simulink model "PV_ESS_MPC_Switching_Template"  (R2025a)
settings: Solver=ode3  StartTime=0.0  StopTime=0.01  FixedStep=Ts_power  RelTol=1e-3
PreLoadFcn:
  | addpath('D:/PV_MPPT/PV_ESS_MPC_Paper_Reproduction/scripts');
model workspace (MAT data in the model file):
  Battery_blocking = 1
  Battery_connect = 0
  Cdc = 0.006
  Cf = 0.001338
  Cpv = 0.005
  Db0 = 0.75
  Db_max = 0.95
  Db_min = 0.05
  Dpv0 = 0.544166666667
  Dpv_max = 0.75
  Dpv_min = 0.35
  Dpv_off_mppt = 0.46
  Dpv_step = 0.0002
  Fsw_bat = 5000
  Fsw_pv = 5000
  G_profile = timeseries
  G_profile.Name = 'unnamed'
  G_profile.DataInfo = tsdata.datametadata
  G_profile.DataInfo.Interpolation = tsdata.interpolation
  G_profile.DataInfo.Interpolation.Fhandle : function handle (value not decoded)
  G_profile.DataInfo.Interpolation.Name = 'linear'
  G_profile.TimeInfo = tsdata.timemetadata
  G_profile.TimeInfo.Length = 5
  G_profile.TimeInfo.DuplicateTimes = 0
  G_profile.TimeInfo.Time_ = [0; 1; 2; 3; 4]
  G_profile.TimeInfo.Initialized = 1
  G_profile.QualityInfo = tsdata.qualmetadata
  G_profile.Data_ = [400; 400; 800; 800; 400]
  GridVpu_profile = timeseries
  GridVpu_profile.Name = 'unnamed'
  GridVpu_profile.DataInfo = tsdata.datametadata
  GridVpu_profile.DataInfo.Interpolation = tsdata.interpolation
  GridVpu_profile.DataInfo.Interpolation.Fhandle : function handle (value not decoded)
  GridVpu_profile.DataInfo.Interpolation.Name = 'linear'
  GridVpu_profile.TimeInfo = tsdata.timemetadata
  GridVpu_profile.TimeInfo.Length = 3
  GridVpu_profile.TimeInfo.DuplicateTimes = 0
  GridVpu_profile.TimeInfo.Time_ = [0; 3.5; 3.500002]
  GridVpu_profile.TimeInfo.Initialized = 1
  GridVpu_profile.QualityInfo = tsdata.qualmetadata
  GridVpu_profile.Data_ = [1; 1; 0.9]
  ILpv0 = 0
  Ibat0 = 0
  Ibat_max = 1666.66666667
  Inverter_connect = 0
  Inverter_enable = 0
  Ki_dc = 200000
  Kii_bat = 0.02
  Kiv_bat = 100
  Kp_dc = 2500
  Kpi_bat = 0.0002
  Kpv_bat = 2
  L_grid_lv = 0.0001
  Lbat = 0.0005
  Lf = 0.0006
  Lpv = 0.0002
  Np_pv = 656
  Ns_pv = 10
  PV_blocking = 1
  PV_connect = 0
  PV_module = 'SunPower SPR-305E-WHT-D'
  P_ac_base = 500000
  P_ac_step = 500000
  P_base_mpc = 2000000
  P_bat_rated = 500000
  P_dc_1 = 600000
  P_dc_2 = 1000000
  P_pv_stc = 2000000
  Pref_max = 2200000
  Pref_min = -2200000
  Q_base_mpc = 1000000
  Q_bat_Ah = 1300
  RLbat = 0.002
  RLpv = 0.002
  R_bat_internal = 0.02
  R_grid_lv = 0.01
  Rdc1_profile = timeseries
  Rdc1_profile.Name = 'unnamed'
  Rdc1_profile.DataInfo = tsdata.datametadata
  Rdc1_profile.DataInfo.Interpolation = tsdata.interpolation
  Rdc1_profile.DataInfo.Interpolation.Fhandle : function handle (value not decoded)
  Rdc1_profile.DataInfo.Interpolation.Name = 'linear'
  Rdc1_profile.TimeInfo = tsdata.timemetadata
  Rdc1_profile.TimeInfo.Length = 3
  Rdc1_profile.TimeInfo.DuplicateTimes = 0
  Rdc1_profile.TimeInfo.Time_ = [0; 1; 1.000002]
  Rdc1_profile.TimeInfo.Initialized = 1
  Rdc1_profile.QualityInfo = tsdata.qualmetadata
  Rdc1_profile.Data_ = [1000000; 1000000; 2.4]
  Rdc2_profile = timeseries
  Rdc2_profile.Name = 'unnamed'
  Rdc2_profile.DataInfo = tsdata.datametadata
  Rdc2_profile.DataInfo.Interpolation = tsdata.interpolation
  Rdc2_profile.DataInfo.Interpolation.Fhandle : function handle (value not decoded)
  Rdc2_profile.DataInfo.Interpolation.Name = 'linear'
  Rdc2_profile.TimeInfo = tsdata.timemetadata
  Rdc2_profile.TimeInfo.Length = 5
  Rdc2_profile.TimeInfo.DuplicateTimes = 0
  Rdc2_profile.TimeInfo.Time_ = [0; 2.5; 2.500002; 3; 3.000002]
  Rdc2_profile.TimeInfo.Initialized = 1
  Rdc2_profile.QualityInfo = tsdata.qualmetadata
  Rdc2_profile.Data_ = [1000000; 1000000; 1.44; 1.44; 1000000]
  Rf = 0.019
  Ron_switch = 0.001
  SOC0 = 50
  SOC_max = 90
  SOC_min = 10
  S_sc_grid = 47000000
  S_tr = 2500000
  T_ac_step = 0.5
  T_dc_1 = 1
  T_dc_2_off = 3
  T_dc_2_on = 2.5
  T_grid_connect = 1.6
  T_grid_dip = 3.5
  T_pv_ramp_down = 3
  T_pv_ramp_up = 1
  T_sync = 1.4
  Ts_bat_ctrl = 0.0001
  Ts_mpc = 5e-05
  Ts_mppt = 0.001
  Ts_power = 2e-06
  V_bat_nom = 300
  V_tr_hv = 25000
  V_tr_lv = 690
  Vac_ll = 690
  Vdc0 = 1200
  Vdc_ref = 1200
  Vf_diode = 1
  Vpv0 = 547
  XR_grid = 10
  f_grid = 50
  lambda_sw = 0.002
  m_var = 4000000
undefined symbols (not defined in the file): DiscIntNeverNeededParam, Ion, Lithium
libraries: spsBreakerLib x5, spsCurrentMeasurementLib x4, spsThreePhaseParallelRLCLoadLib x3, spsThreePhaseVIMeasurementLib x3, spsThreePhaseBreakerLib x2, spsPWMGeneratorDCDCLib x2, spsParallelRLCBranchLib x2, spsVariableResistorLib x2, spsSeriesRLCBranchLib x2, spsVoltageMeasurementLib x2, spsBatteryLib x1, spsTwoQuadrantDCDCConverterLib x1
settings Model: Creator=Limingyu  LastModifiedBy=Limingyu
settings DataIOCC: SignalLogging=off

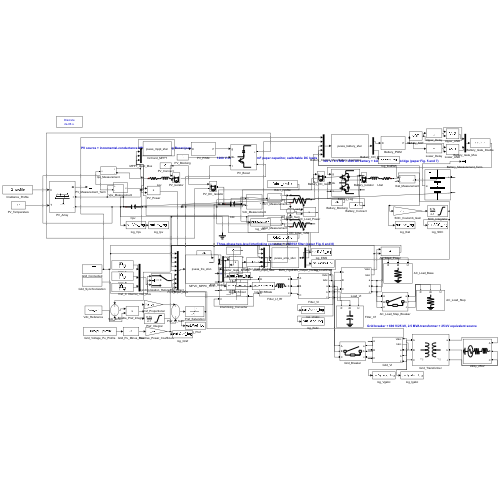
[thumbnail: Simulink's stored preview of the top-level diagram]
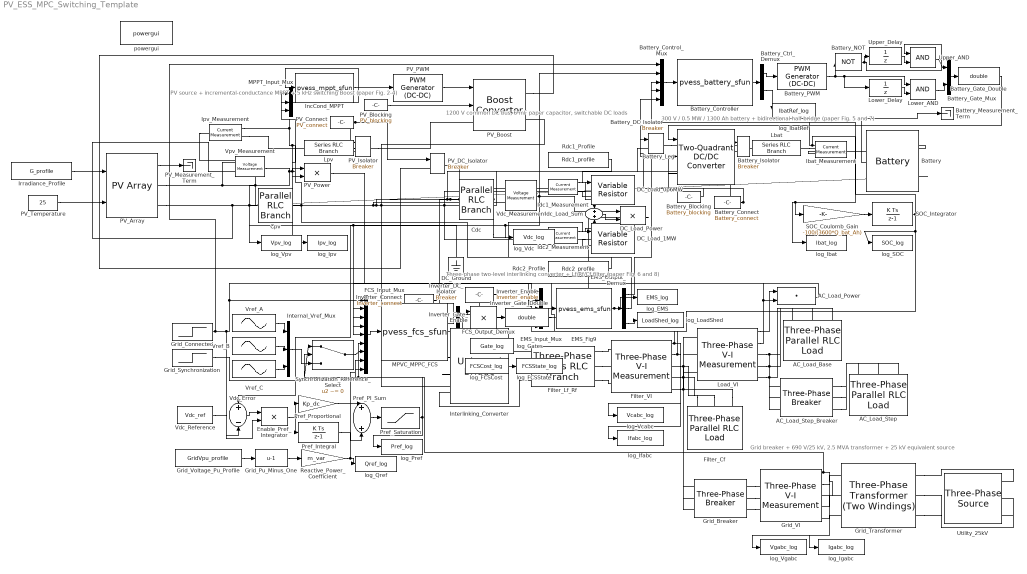
== system PV_ESS_MPC_Switching_Template ==
  note: PV source + incremental-conductance MPPT + 5 kHz switching Boost (paper Fig. 2-4)
  note: 1200 V common DC bus, 6 mF paper capacitor, switchable DC loads
  note: 300 V / 0.5 MW / 1300 Ah battery + bidirectional half bridge (paper Fig. 5 and 7)
  note: Three-phase two-level interlinking converter + Lf/Rf/Cf filter (paper Fig. 6 and 8)
  note: Grid breaker + 690 V/25 kV, 2.5 MVA transformer + 25 kV equivalent source
  AC_Load_Base : spsThreePhaseParallelRLCLoadLib/Three-Phase Parallel RLC Load  LConnTagsString=A|B|C  Configuration=Y (grounded)  NominalVoltage=Vac_ll  Vabc=[1e3 1e3 1e3]  Vabcp=[1e3 1e3 1e3]  NominalFrequency=f_grid  UnbalancedPower=off  ActivePower=P_ac_base  InductivePower=0  CapacitivePower=0  Pabc=[10e3 9e3 11e3]  QLabc=[100 90 110]  QCabc=[100 90 110]  Pabcp=[10e3 9e3 11e3]  QLabcp=[100 90 110]  QCabcp=[100 90 110]  Measurements=None  LoadType=constant Z
  AC_Load_Power : DotProduct  OutDataTypeStr=Inherit: Inherit via internal rule
  AC_Load_Step : spsThreePhaseParallelRLCLoadLib/Three-Phase Parallel RLC Load  LConnTagsString=A|B|C  Configuration=Y (grounded)  NominalVoltage=Vac_ll  Vabc=[1e3 1e3 1e3]  Vabcp=[1e3 1e3 1e3]  NominalFrequency=f_grid  UnbalancedPower=off  ActivePower=P_ac_step  InductivePower=0  CapacitivePower=0  Pabc=[10e3 9e3 11e3]  QLabc=[100 90 110]  QCabc=[100 90 110]  Pabcp=[10e3 9e3 11e3]  QLabcp=[100 90 110]  QCabcp=[100 90 110]  Measurements=None  LoadType=constant Z
  AC_Load_Step_Breaker : spsThreePhaseBreakerLib/Three-Phase Breaker  InitialState=open  SwitchA=on  SwitchB=on  SwitchC=on  SwitchTimes=T_ac_step  External=off  BreakerResistance=1e-3  SnubberResistance=1e6  SnubberCapacitance=inf  Measurements=None
  Battery : spsBatteryLib/Battery  BatType=Lithium-Ion  NomV=V_bat_nom  NomQ=Q_bat_Ah  SOC=SOC0  Batt_Tr=1  PresetModel=off  MaxQ=Q_bat_Ah  MinV=270  FullV=330  Dis_rate=650  R=R_bat_internal  Normal_OP=1170  expZone=[315,65]
  Battery_Blocking : Constant  Value=Battery_blocking
  Battery_Connect : Constant  Value=Battery_connect
  Battery_Control_Mux : Mux  Inputs=5
  Battery_Controller : M-S-Function  FunctionName=pvess_battery_sfun  Parameters=Ts_bat_ctrl,Vdc_ref,SOC_min,SOC_max,Ibat_max,Kpv_bat,Kiv_bat,Kpi_bat,Kii_bat,V_bat_nom,Db_min,Db_max
  Battery_Ctrl_Demux : Demux  Outputs=[1 1]
  Battery_DC_Isolator : spsBreakerLib/Breaker  InitialState=1  SwitchingTimes="[1/60  5/60]"  External=on  BreakerResistance=1e-3  SnubberResistance=1e6  SnubberCapacitance=inf  Measurements=None  MoreParameters=on  NoBreakLoop=off
  Battery_Gate_Double : DataTypeConversion  OutDataTypeStr=double  SaturateOnIntegerOverflow=off  RndMeth=Floor
  Battery_Gate_Mux : Mux  Inputs=2
  Battery_Isolator : spsBreakerLib/Breaker  InitialState=1  SwitchingTimes="[1/60  5/60]"  External=on  BreakerResistance=1e-3  SnubberResistance=1e6  SnubberCapacitance=inf  Measurements=None  MoreParameters=on  NoBreakLoop=off
  Battery_Leg : spsTwoQuadrantDCDCConverterLib/Two-Quadrant DC//DC Converter  ModelType=Switching devices  Ron=Ron_switch  Rs=1e6  Cs=inf  Vforward=[0,0]  Ron_Diode=Ron_switch  Rs_Diode=1e6  Cs_Diode=inf  Vf_Diode=0  Rs_CurrentSource=inf  Ron_ACsource=1e-3
  Battery_Measurement_Term : Terminator
  Battery_NOT : Logic  Operator=NOT  AllPortsSameDT=off  OutDataTypeStr=boolean
  Battery_PWM : spsPWMGeneratorDCDCLib/PWM Generator (DC-DC)  Fsw=Fsw_bat  Ts=Ts_power
  Cdc : spsParallelRLCBranchLib/Parallel RLC Branch  LConnTagsString=a  RConnTagsString=__new0  BranchType=C  Resistance=1  Inductance=1e-3  SetiL0=off  InitialCurrent=0  Capacitance=Cdc  Setx0=on  InitialVoltage=Vdc0  Measurements=None
  Cpv : spsParallelRLCBranchLib/Parallel RLC Branch  LConnTagsString=a  RConnTagsString=__new0  BranchType=C  Resistance=1  Inductance=1e-3  SetiL0=off  InitialCurrent=0  Capacitance=Cpv  Setx0=on  InitialVoltage=Vpv0  Measurements=None
  DC_Ground : spsGroundLib/Ground  LConnTagsString=a
  DC_Load_0p6MW : spsVariableResistorLib/Variable Resistor  Rabsmin=0.2
  DC_Load_1MW : spsVariableResistorLib/Variable Resistor  Rabsmin=0.2
  DC_Load_Power : Product
  EMS_Fig9 : M-S-Function  FunctionName=pvess_ems_sfun  Parameters=SOC_min,SOC_max
  EMS_Input_Mux : Mux  Inputs=5
  EMS_Output_Demux : Demux  Outputs=3
  Enable_Pref_Integrator : Product
  FCS_Input_Mux : Mux  Inputs=9
  FCS_Output_Demux : Demux  Outputs=[6 1 1]
  Filter_Cf : spsThreePhaseParallelRLCLoadLib/Three-Phase Parallel RLC Load  LConnTagsString=A|B|C  Configuration=Y (grounded)  NominalVoltage=Vac_ll  Vabc=[1e3 1e3 1e3]  Vabcp=[1e3 1e3 1e3]  NominalFrequency=f_grid  UnbalancedPower=off  ActivePower=0  InductivePower=0  CapacitivePower=2*pi*f_grid*Cf*Vac_ll^2  Pabc=[10e3 9e3 11e3]  QLabc=[100 90 110]  QCabc=[100 90 110]  Pabcp=[10e3 9e3 11e3]  QLabcp=[100 90 110]  QCabcp=[100 90 110]  Measurements=None  LoadType=constant Z
  Filter_Lf_Rf : spsThreePhaseSeriesRLCBranchLib/Three-Phase Series RLC Branch  LConnTagsString=A|B|C  RConnTagsString=A|B|C  BranchType=RL  Resistance=Rf  Inductance=Lf  Capacitance=1e-6  Measurements=None
  Filter_VI : spsThreePhaseVIMeasurementLib/Three-Phase V-I Measurement  VoltageMeasurement=phase-to-ground  SetLabelV=off  LabelV=Vabc  Vpu=off  VpuLL=off  CurrentMeasurement=yes  SetLabelI=off  LabelI=Iabc  Ipu=off  Pbase=100e6  Vbase=500e3  OutputType=Complex  PhasorSimulation=off  PSBequivalent=0
  Grid_Breaker : spsThreePhaseBreakerLib/Three-Phase Breaker  InitialState=open  SwitchA=on  SwitchB=on  SwitchC=on  SwitchTimes=T_grid_connect  External=off  BreakerResistance=1e-3  SnubberResistance=1e6  SnubberCapacitance=inf  Measurements=None
  Grid_Connected : Step  Time=T_grid_connect  SampleTime=Ts_mpc
  Grid_Pu_Minus_One : Bias  Bias=-1  SaturateOnIntegerOverflow=off
  Grid_Synchronization : Step  Time=T_sync  SampleTime=Ts_mpc
  Grid_Transformer : spsThreePhaseTransformerTwoWindingsLib/Three-Phase Transformer (Two Windings)  Winding1Connection=Yg  Winding2Connection=Yg  CoreType=Three single-phase transformers  SetSaturation=off  Hysteresis=off  DataFile='hysteresis'  SetInitialFlux=off  Measurements=None  UNITS=pu  NominalPower=[S_tr,f_grid]  Winding1=[V_tr_lv,0.002,0.06]  Winding2=[V_tr_hv,0.002,0.06]  Rm=500  Lm=500  L0=0.5  Saturation=[ 0,0 ; 0.0024,1.2 ; 1.0,1.52 ]  InitialFluxes=[ 0.8 , -0.8 , 0.7 ]  BreakLoop=off  DiscreteSolver=Trapezoidal iterative  DataType=off  TransfoNumber=1
  Grid_VI : spsThreePhaseVIMeasurementLib/Three-Phase V-I Measurement  VoltageMeasurement=phase-to-ground  SetLabelV=off  LabelV=Vabc  Vpu=off  VpuLL=off  CurrentMeasurement=yes  SetLabelI=off  LabelI=Iabc  Ipu=off  Pbase=100e6  Vbase=500e3  OutputType=Complex  PhasorSimulation=off  PSBequivalent=0
  Grid_Voltage_Pu_Profile : FromWorkspace  VariableName=GridVpu_profile
  Ibat_Measurement : spsCurrentMeasurementLib/Current Measurement  PhasorSimulation=off  OutputType=Complex  PSBequivalent=0
  Idc1_Measurement : spsCurrentMeasurementLib/Current Measurement  PhasorSimulation=off  OutputType=Complex  PSBequivalent=0
  Idc2_Measurement : spsCurrentMeasurementLib/Current Measurement  PhasorSimulation=off  OutputType=Complex  PSBequivalent=0
  Idc_Load_Sum : Sum
  IncCond_MPPT : M-S-Function  FunctionName=pvess_mppt_sfun  Parameters=Ts_mppt,Dpv0,Dpv_min,Dpv_max,Dpv_step,Dpv_off_mppt
  Interlinking_Converter : spsUniversalBridgeLib/Universal Bridge  Arms=3  SnubberResistance=1e5  SnubberCapacitance=inf  Device=IGBT / Diodes  Ron=Ron_switch  Lon=0  ForwardVoltages=[Vf_diode,Vf_diode]  ForwardVoltage=0  GTOparameters=[ 10e-6 , 20e-6 ]  IGBTparameters=[ 1e-6 , 2e-6 ]  Measurements=None  Measurements_2=None  converterType=Rectifier
  Internal_Vref_Mux : Mux  Inputs=3
  Inverter_Connect : Constant  Value=Inverter_connect
  Inverter_DC_Isolator : spsBreakerLib/Breaker  InitialState=1  SwitchingTimes="[1/60  5/60]"  External=on  BreakerResistance=1e-3  SnubberResistance=1e6  SnubberCapacitance=inf  Measurements=None  MoreParameters=on  NoBreakLoop=off
  Inverter_Enable : Constant  Value=Inverter_enable
  Inverter_Gate_Double : DataTypeConversion  OutDataTypeStr=double  SaturateOnIntegerOverflow=off  RndMeth=Floor
  Inverter_Gate_Enable : Product
  Ipv_Measurement : spsCurrentMeasurementLib/Current Measurement  PhasorSimulation=off  OutputType=Complex  PSBequivalent=0
  Irradiance_Profile : FromWorkspace  VariableName=G_profile
  Lbat : spsSeriesRLCBranchLib/Series RLC Branch  LConnTagsString=__new0  RConnTagsString=__new0  BranchType=RL  Resistance=RLbat  Inductance=Lbat  SetiL0=on  InitialCurrent=Ibat0  Capacitance=1e-6  Setx0=off  InitialVoltage=0  Measurements=None
  Load_VI : spsThreePhaseVIMeasurementLib/Three-Phase V-I Measurement  VoltageMeasurement=phase-to-ground  SetLabelV=off  LabelV=Vabc  Vpu=off  VpuLL=off  CurrentMeasurement=yes  SetLabelI=off  LabelI=Iabc  Ipu=off  Pbase=100e6  Vbase=500e3  OutputType=Complex  PhasorSimulation=off  PSBequivalent=0
  Lower_AND : Logic  AllPortsSameDT=off  OutDataTypeStr=boolean
  Lower_Delay : UnitDelay  SampleTime=Ts_power  HasFrameUpgradeWarning=on
  Lpv : spsSeriesRLCBranchLib/Series RLC Branch  LConnTagsString=__new0  RConnTagsString=__new0  BranchType=RL  Resistance=RLpv  Inductance=Lpv  SetiL0=on  InitialCurrent=ILpv0  Capacitance=1e-6  Setx0=off  InitialVoltage=0  Measurements=None
  MPPT_Input_Mux : Mux  Inputs=3
  MPVC_MPPC_FCS : M-S-Function  FunctionName=pvess_fcs_sfun  Parameters=Ts_mpc,Lf,Cf,Rf,P_base_mpc,Q_base_mpc,lambda_sw
  PV_Array : spsPVArrayLib/PV Array  Npar=Np_pv  Nser=Ns_pv  PlotType=array @ 1000 W/m2 & specified temperatures  S_vec="[ 1000  500  100 ]"  Temp_C_vec="[ 45 25  ]"  ModuleName=SunPower SPR-305E-WHT-D  PlotWhenSelected=off  Pm=305.226  Ncell=96  Voc=64.2  Isc=5.96  Vm=54.7  Im=5.58  beta_Voc_pc=-0.2727  alpha_Isc_pc=0.061745  beta_Voc=-0.17507  alpha_Isc=0.00368  IL=5.9657  I0=6.3076e-12  nI=0.94489  Rsh=393.2054  Rs=0.37428  RobustModel=off  RobustCellTemperature=313.3991  BAL=on  Tc=Ts_power  Tfilter=5e-5
  PV_Blocking : Constant  Value=PV_blocking
  PV_Boost : spsBoostConverterLib/Boost Converter  ModelType=Switching devices  Ron=Ron_switch  Rs=1e6  Cs=inf  Vforward=[0,0]  Ron_Diode=Ron_switch  Rs_Diode=1e6  Cs_Diode=inf  Vf_Diode=Vf_diode  Rs_CurrentSource=inf  Ron_ACsource=1e-3
  PV_Connect : Constant  Value=PV_connect
  PV_DC_Isolator : spsBreakerLib/Breaker  InitialState=1  SwitchingTimes="[1/60  5/60]"  External=on  BreakerResistance=1e-3  SnubberResistance=1e6  SnubberCapacitance=inf  Measurements=None  MoreParameters=on  NoBreakLoop=off
  PV_Isolator : spsBreakerLib/Breaker  InitialState=1  SwitchingTimes="[1/60  5/60]"  External=on  BreakerResistance=1e-3  SnubberResistance=1e6  SnubberCapacitance=inf  Measurements=None  MoreParameters=on  NoBreakLoop=off
  PV_Measurement_Term : Terminator
  PV_PWM : spsPWMGeneratorDCDCLib/PWM Generator (DC-DC)  Fsw=Fsw_pv  Ts=Ts_power
  PV_Power : Product
  PV_Temperature : Constant  Value=25
  Pref_Integral : DiscreteIntegrator  gainval=Ki_dc  SampleTime=Ts_mpc  LimitOutput=on  UpperSaturationLimit=Pref_max  LowerSaturationLimit=Pref_min  ICPrevOutput=DiscIntNeverNeededParam  ICPrevScaledInput=DiscIntNeverNeededParam
  Pref_PI_Sum : Sum
  Pref_Proportional : Gain  Gain=Kp_dc
  Pref_Saturation : Saturate  UpperLimit=Pref_max  LowerLimit=Pref_min
  Rdc1_Profile : FromWorkspace  VariableName=Rdc1_profile
  Rdc2_Profile : FromWorkspace  VariableName=Rdc2_profile
  Reactive_Power_Coefficient : Gain  Gain=m_var
  SOC_Coulomb_Gain : Gain  Gain=-100/(3600*Q_bat_Ah)
  SOC_Integrator : DiscreteIntegrator  gainval=1  InitialCondition=SOC0  SampleTime=Ts_bat_ctrl  LimitOutput=on  UpperSaturationLimit=100  LowerSaturationLimit=0  ICPrevOutput=DiscIntNeverNeededParam  ICPrevScaledInput=DiscIntNeverNeededParam
  Synchronization_Reference_Select : Switch  Criteria=u2 ~= 0  Threshold=0.5  SaturateOnIntegerOverflow=off  InputSameDT=off
  Upper_AND : Logic  AllPortsSameDT=off  OutDataTypeStr=boolean
  Upper_Delay : UnitDelay  SampleTime=Ts_power  HasFrameUpgradeWarning=on
  Utility_25kV : spsThreePhaseSourceLib/Three-Phase Source  InternalConnection=Yg  VoltagePhases=off  Voltage=V_tr_hv  PhaseAngle=0  Voltage_phases=[25e3 25e3 25e3]/sqrt(3)  PhaseAngles_phases=[0 -120 +120]  Frequency=f_grid  NonIdealSource=on  SpecifyImpedance=off  Resistance=0.8929  Inductance=16.58e-3  ShortCircuitLevel=S_sc_grid  BaseVoltage=V_tr_hv  XRratio=XR_grid  BusType=swing  Pref=10e3  Qref=0  Prefabc=[10e3, 10e3, 10e3]  Qrefabc=[0, 0, 0]  Qmin=-inf  Qmax=inf
  Vdc_Error : Sum  Inputs=+-
  Vdc_Measurement : spsVoltageMeasurementLib/Voltage Measurement  PhasorSimulation=off  OutputType=Complex  PSBequivalent=0
  Vdc_Reference : Constant  Value=Vdc_ref
  Vpv_Measurement : spsVoltageMeasurementLib/Voltage Measurement  PhasorSimulation=off  OutputType=Complex  PSBequivalent=0
  Vref_A : Sin  Amplitude=sqrt(2)*Vac_ll/sqrt(3)  Frequency=2*pi*f_grid  SampleTime=Ts_mpc
  Vref_B : Sin  Amplitude=sqrt(2)*Vac_ll/sqrt(3)  Frequency=2*pi*f_grid  Phase=-2*pi/3  SampleTime=Ts_mpc
  Vref_C : Sin  Amplitude=sqrt(2)*Vac_ll/sqrt(3)  Frequency=2*pi*f_grid  Phase=2*pi/3  SampleTime=Ts_mpc
  log_EMS : ToWorkspace  VariableName=EMS_log  SaveFormat=Timeseries  SampleTime=-1
  log_FCSCost : ToWorkspace  VariableName=FCSCost_log  SaveFormat=Timeseries  SampleTime=-1
  log_FCSState : ToWorkspace  VariableName=FCSState_log  SaveFormat=Timeseries  SampleTime=-1
  log_Gates : ToWorkspace  VariableName=Gate_log  SaveFormat=Timeseries  SampleTime=-1
  log_Ibat : ToWorkspace  VariableName=Ibat_log  SaveFormat=Timeseries  SampleTime=-1
  log_IbatRef : ToWorkspace  VariableName=IbatRef_log  SaveFormat=Timeseries  SampleTime=-1
  log_Ifabc : ToWorkspace  VariableName=Ifabc_log  SaveFormat=Timeseries  SampleTime=-1
  log_Igabc : ToWorkspace  VariableName=Igabc_log  SaveFormat=Timeseries  SampleTime=-1
  log_Ipv : ToWorkspace  VariableName=Ipv_log  SaveFormat=Timeseries  SampleTime=-1
  log_LoadShed : ToWorkspace  VariableName=LoadShed_log  SaveFormat=Timeseries  SampleTime=-1
  log_Pref : ToWorkspace  VariableName=Pref_log  SaveFormat=Timeseries  SampleTime=-1
  log_Qref : ToWorkspace  VariableName=Qref_log  SaveFormat=Timeseries  SampleTime=-1
  log_SOC : ToWorkspace  VariableName=SOC_log  SaveFormat=Timeseries  SampleTime=-1
  log_Vcabc : ToWorkspace  VariableName=Vcabc_log  SaveFormat=Timeseries  SampleTime=-1
  log_Vdc : ToWorkspace  VariableName=Vdc_log  SaveFormat=Timeseries  SampleTime=-1
  log_Vgabc : ToWorkspace  VariableName=Vgabc_log  SaveFormat=Timeseries  SampleTime=-1
  log_Vpv : ToWorkspace  VariableName=Vpv_log  SaveFormat=Timeseries  SampleTime=-1
  powergui : spspowerguiLib/powergui  Priority=1  SimulationMode=Discrete  SampleTime=Ts_power  frequency=60  Iterations=50  frequencyindice=60  Pbase=100e6  ErrMax=1e-4  UnitsV=kV  UnitsW=MW  buscounter=0  FunctionMessages=off  echomessages=off  EnableUseOfTLC=off  CurrentSourceSwitches=off  DisableSnubberDevices=off  DisableRonSwitches=off  DisableVfSwitches=off  DisplayEquations=off  AutomaticDiscreteSolvers=off  SolverType=Tustin/Backward Euler (TBE)  Interpol=off  ExternalGateDelay=off  methode=off  Ts=100  x0status=blocks  SPID=on  SwTol=0  HookPort=off  NonlinearTolerance=1e-4  nMaxIteration=100  ContinueOnMaxIteration=off  RestoreLinks=warning  ResistiveCurrentMeasurement=off  Frange=[0:2:500]  Ylog=off  Xlog=on  ShowGrid=off  save=off  variable=ZData  structure=0  ZoomFFT=off  StartTime=0.0  cycles=1  DisplayStyle=1  fundamental=60  FreqAxis=off  MaxFrequency=1000  frequencyindicesteady=1  RmsSteady=1  display=off
  wires:
  Irradiance_Profile/1 -> PV_Array/1
  PV_Temperature/1 -> PV_Array/2
  PV_Array/1 -> PV_Measurement_Term/1
  Vpv_Measurement/1 -> MPPT_Input_Mux/1, PV_Power/1, log_Vpv/1
  Ipv_Measurement/1 -> PV_Power/2, log_Ipv/1, MPPT_Input_Mux/2
  EMS_Output_Demux/2 -> MPPT_Input_Mux/3
  MPPT_Input_Mux/1 -> IncCond_MPPT/1
  IncCond_MPPT/1 -> PV_PWM/1
  PV_PWM/1 -> PV_Boost/1
  PV_Blocking/1 -> PV_Boost/2
  PV_Connect/1 -> PV_Isolator/1, PV_DC_Isolator/1
  Rdc1_Profile/1 -> DC_Load_0p6MW/1
  Rdc2_Profile/1 -> DC_Load_1MW/1
  Idc1_Measurement/1 -> Idc_Load_Sum/1
  Idc2_Measurement/1 -> Idc_Load_Sum/2
  Vdc_Measurement/1 -> Vdc_Error/1, FCS_Input_Mux/2, log_Vdc/1, DC_Load_Power/1, Battery_Control_Mux/2
  Idc_Load_Sum/1 -> DC_Load_Power/2
  Battery/1 -> Battery_Measurement_Term/1
  Ibat_Measurement/1 -> SOC_Coulomb_Gain/1, log_Ibat/1, Battery_Control_Mux/3
  SOC_Coulomb_Gain/1 -> SOC_Integrator/1
  Grid_Connected/1 -> FCS_Input_Mux/1, EMS_Input_Mux/1, Enable_Pref_Integrator/2, Battery_Control_Mux/1
  SOC_Integrator/1 -> EMS_Input_Mux/5, log_SOC/1, Battery_Control_Mux/4
  EMS_Output_Demux/1 -> Battery_Control_Mux/5
  Battery_Control_Mux/1 -> Battery_Controller/1
  Battery_Controller/1 -> Battery_Ctrl_Demux/1
  Battery_Ctrl_Demux/1 -> Battery_PWM/1
  Battery_Ctrl_Demux/2 -> log_IbatRef/1
  Battery_PWM/1 -> Lower_Delay/1, Lower_AND/1, Battery_NOT/1
  Battery_NOT/1 -> Upper_Delay/1, Upper_AND/1
  Upper_Delay/1 -> Upper_AND/2
  Lower_Delay/1 -> Lower_AND/2
  Upper_AND/1 -> Battery_Gate_Mux/1
  Lower_AND/1 -> Battery_Gate_Mux/2
  Battery_Gate_Mux/1 -> Battery_Gate_Double/1
  Battery_Gate_Double/1 -> Battery_Leg/1
  Battery_Blocking/1 -> Battery_Leg/2
  Battery_Connect/1 -> Battery_Isolator/1, Battery_DC_Isolator/1
  Vref_A/1 -> Internal_Vref_Mux/1
  Vref_B/1 -> Internal_Vref_Mux/2
  Vref_C/1 -> Internal_Vref_Mux/3
  Grid_VI/1 -> Synchronization_Reference_Select/1, FCS_Input_Mux/6, log_Vgabc/1
  Grid_Synchronization/1 -> Synchronization_Reference_Select/2
  Internal_Vref_Mux/1 -> Synchronization_Reference_Select/3
  Vdc_Reference/1 -> Vdc_Error/2
  Vdc_Error/1 -> Enable_Pref_Integrator/1
  Enable_Pref_Integrator/1 -> Pref_Proportional/1, Pref_Integral/1
  Pref_Proportional/1 -> Pref_PI_Sum/1
  Pref_Integral/1 -> Pref_PI_Sum/2
  Pref_PI_Sum/1 -> Pref_Saturation/1
  Grid_Voltage_Pu_Profile/1 -> Grid_Pu_Minus_One/1
  Grid_Pu_Minus_One/1 -> Reactive_Power_Coefficient/1
  Filter_VI/1 -> FCS_Input_Mux/3, log_Vcabc/1
  Filter_VI/2 -> FCS_Input_Mux/4, log_Ifabc/1
  Load_VI/2 -> FCS_Input_Mux/5, AC_Load_Power/2
  Synchronization_Reference_Select/1 -> FCS_Input_Mux/7
  Pref_Saturation/1 -> FCS_Input_Mux/8, log_Pref/1
  Reactive_Power_Coefficient/1 -> FCS_Input_Mux/9, log_Qref/1
  FCS_Input_Mux/1 -> MPVC_MPPC_FCS/1
  MPVC_MPPC_FCS/1 -> FCS_Output_Demux/1
  FCS_Output_Demux/1 -> Inverter_Gate_Enable/1, log_Gates/1
  Inverter_Enable/1 -> Inverter_Gate_Enable/2
  Inverter_Connect/1 -> Inverter_DC_Isolator/1
  Inverter_Gate_Enable/1 -> Inverter_Gate_Double/1
  Inverter_Gate_Double/1 -> Interlinking_Converter/1
  Load_VI/1 -> AC_Load_Power/1
  PV_Power/1 -> EMS_Input_Mux/2
  AC_Load_Power/1 -> EMS_Input_Mux/3
  DC_Load_Power/1 -> EMS_Input_Mux/4
  EMS_Input_Mux/1 -> EMS_Fig9/1
  EMS_Fig9/1 -> EMS_Output_Demux/1, log_EMS/1
  Grid_VI/2 -> log_Igabc/1
  FCS_Output_Demux/2 -> log_FCSCost/1
  FCS_Output_Demux/3 -> log_FCSState/1
  EMS_Output_Demux/3 -> log_LoadShed/1
  connections:
  Ipv_Measurement/LConn1 -- PV_Array/RConn1 -- Vpv_Measurement/LConn1 -- Cpv/LConn1
  Ipv_Measurement/RConn1 -- Lpv/LConn1
  Lpv/RConn1 -- PV_Isolator/LConn1
  PV_Isolator/RConn1 -- PV_Boost/LConn1
  Cpv/RConn1 -- PV_Boost/RConn2 -- DC_Load_0p6MW/RConn1 -- DC_Load_1MW/RConn1 -- Battery_Leg/RConn2 -- Interlinking_Converter/RConn2 -- Cdc/RConn1 -- Vdc_Measurement/LConn2 -- PV_Array/RConn2 -- Vpv_Measurement/LConn2 -- DC_Ground/LConn1 -- Battery/LConn2
  PV_Boost/RConn1 -- PV_DC_Isolator/LConn1
  PV_DC_Isolator/RConn1 -- Idc2_Measurement/LConn1 -- Idc1_Measurement/LConn1 -- Vdc_Measurement/LConn1 -- Inverter_DC_Isolator/LConn1 -- Battery_DC_Isolator/LConn1 -- Cdc/LConn1
  Battery_DC_Isolator/RConn1 -- Battery_Leg/RConn1
  Inverter_DC_Isolator/RConn1 -- Interlinking_Converter/RConn1
  Idc1_Measurement/RConn1 -- DC_Load_0p6MW/LConn1
  Idc2_Measurement/RConn1 -- DC_Load_1MW/LConn1
  Battery_Leg/LConn1 -- Battery_Isolator/LConn1
  Battery_Isolator/RConn1 -- Lbat/RConn1
  Lbat/LConn1 -- Ibat_Measurement/RConn1
  Ibat_Measurement/LConn1 -- Battery/LConn1
  Interlinking_Converter/LConn1 -- Filter_Lf_Rf/LConn1
  Filter_Lf_Rf/RConn1 -- Filter_VI/LConn1
  Filter_Cf/LConn1 -- Filter_VI/RConn1 -- Load_VI/LConn1 -- Grid_Breaker/LConn1
  AC_Load_Base/LConn1 -- Load_VI/RConn1 -- AC_Load_Step_Breaker/LConn1
  AC_Load_Step_Breaker/RConn1 -- AC_Load_Step/LConn1
  Grid_Breaker/RConn1 -- Grid_VI/LConn1
  Grid_VI/RConn1 -- Grid_Transformer/LConn1
  Grid_Transformer/RConn1 -- Utility_25kV/RConn1
  Interlinking_Converter/LConn2 -- Filter_Lf_Rf/LConn2
  Filter_Lf_Rf/RConn2 -- Filter_VI/LConn2
  Filter_Cf/LConn2 -- Filter_VI/RConn2 -- Load_VI/LConn2 -- Grid_Breaker/LConn2
  AC_Load_Base/LConn2 -- Load_VI/RConn2 -- AC_Load_Step_Breaker/LConn2
  AC_Load_Step_Breaker/RConn2 -- AC_Load_Step/LConn2
  Grid_Breaker/RConn2 -- Grid_VI/LConn2
  Grid_VI/RConn2 -- Grid_Transformer/LConn2
  Grid_Transformer/RConn2 -- Utility_25kV/RConn2
  Interlinking_Converter/LConn3 -- Filter_Lf_Rf/LConn3
  Filter_Lf_Rf/RConn3 -- Filter_VI/LConn3
  Filter_Cf/LConn3 -- Filter_VI/RConn3 -- Load_VI/LConn3 -- Grid_Breaker/LConn3
  AC_Load_Base/LConn3 -- Load_VI/RConn3 -- AC_Load_Step_Breaker/LConn3
  AC_Load_Step_Breaker/RConn3 -- AC_Load_Step/LConn3
  Grid_Breaker/RConn3 -- Grid_VI/LConn3
  Grid_VI/RConn3 -- Grid_Transformer/LConn3
  Grid_Transformer/RConn3 -- Utility_25kV/RConn3
